simulink model "BiomT1_NOPROP_Model"  (R2023b)
settings: Solver=VariableStepAuto  StartTime=0.0  StopTime=100.0  RelTol=1e-3
values from neighbouring files (symbols this model uses):
  g = 9.81    [initialize_model.m]
  inertiaGeom = load_inertiaGeom()    [computeAeroFM.m]    (also in initialize_model.m)
  x0 = [0 0 zbar u0 v0 w0 0 0 0 0 0 0]    [FlightPerf.m]    (also in initialize_model.m)
libraries: aerolibasang x2, shared6dof x1, aerolibatmos2 x1
settings Model: Creator=sherpa  LastModifiedBy=sudip
settings SolverCC: AlgebraicLoopSolver=TrustRegion
settings OptimizationCC: ReuseModelBlockBuffer=off
settings DebuggingCC: UnconnectedInputMsg=warning  UnconnectedOutputMsg=warning  UnconnectedLineMsg=warning
settings ModelReferenceCC: EnableRefExpFcnMdlSchedulingChecks=on
settings RTWCC: DLArmComputeVersion=19.05

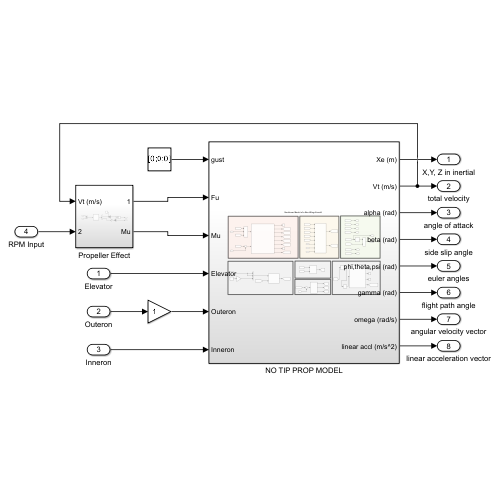
[thumbnail: Simulink's stored preview of the top-level diagram]
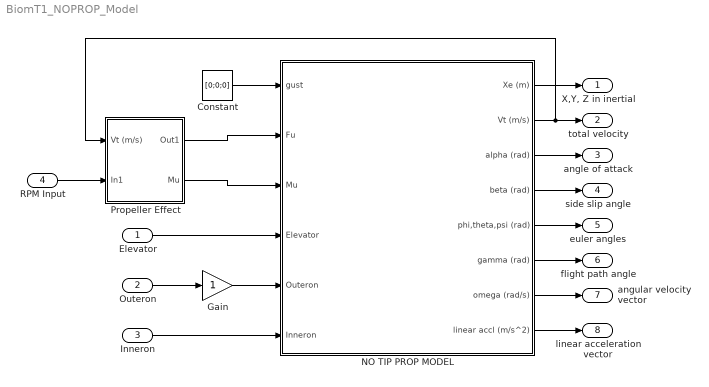
== system BiomT1_NOPROP_Model ==
  Elevator : Inport
  Outeron : Inport  Port=2
  Inneron : Inport  Port=3
  RPM Input : Inport  Port=4
  Constant : Constant  Value=[0;0;0]
  Gain : Gain
  NO TIP PROP MODEL : Subsystem
  Propeller Effect : Subsystem
  "X,Y, Z in inertial" : Outport
  total velocity : Outport  Port=2
  angle of attack : Outport  Port=3
  side slip angle : Outport  Port=4
  euler angles : Outport  Port=5
  flight path angle : Outport  Port=6
  angular velocity vector : Outport  Port=7
  linear acceleration vector : Outport  Port=8
  wires:
  NO TIP PROP MODEL/1(Xe (m)) -> "X,Y, Z in inertial"/1
  NO TIP PROP MODEL/2(Vt (m/s)) -> Propeller Effect/1(Vt (m/s)), total velocity/1
  NO TIP PROP MODEL/3(alpha (rad)) -> angle of attack/1
  NO TIP PROP MODEL/4(beta (rad)) -> side slip angle/1
  NO TIP PROP MODEL/6(gamma (rad)) -> flight path angle/1
  NO TIP PROP MODEL/7(omega (rad/s)) -> angular velocity vector/1
  NO TIP PROP MODEL/8(linear accl (m/s^2)) -> linear acceleration vector/1
  NO TIP PROP MODEL/5(phi,theta,psi (rad)) -> euler angles/1
  Constant/1 -> NO TIP PROP MODEL/1(gust)
  Outeron/1 -> Gain/1
  Inneron/1 -> NO TIP PROP MODEL/6(Inneron)
  Propeller Effect/1(Out1) -> NO TIP PROP MODEL/2(Fu)
  RPM Input/1 -> Propeller Effect/2(In1)
  Propeller Effect/2(Mu) -> NO TIP PROP MODEL/3(Mu)
  Gain/1 -> NO TIP PROP MODEL/5(Outeron)
  Elevator/1 -> NO TIP PROP MODEL/4("Elevator ")

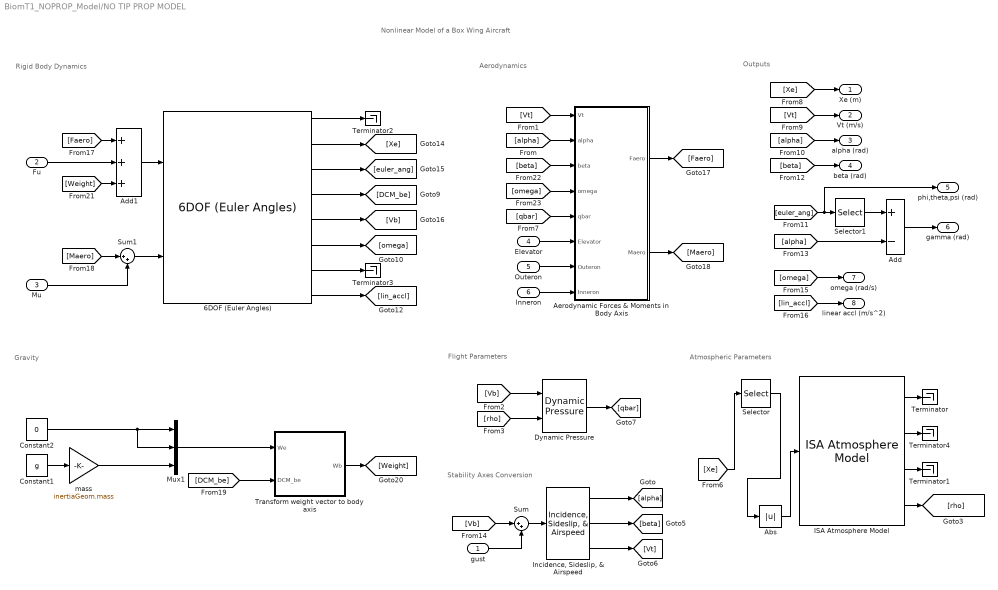
== system BiomT1_NOPROP_Model/NO TIP PROP MODEL ==
  note: Gravity
  note: Nonlinear Model of a Box Wing Aircraft
  note: Aerodynamics
  note: Outputs
  note: Rigid Body Dynamics
  note: Stability Axes Conversion
  note: Atmospheric Parameters
  note: Flight Parameters
  gust : Inport  PortDimensions=3
  Fu : Inport  Port=2  PortDimensions=3
  Mu : Inport  Port=3  PortDimensions=3
  "Elevator " : Inport  Port=4
  Outeron : Inport  Port=5
  Inneron : Inport  Port=6
  6DOF (Euler Angles) : shared6dof/6DOF (Euler Angles)  units=Metric (MKS)  mtype=Fixed  rep=Euler Angles  xme_0=x0(1:3)  Vm_0=x0(4:6)  eul_0=x0(7:9)  pm_0=x0(10:12)  mass_0=inertiaGeom.mass  mass_e=0.5  mass_f=2.0  inertia=inertiaGeom.inertiaMatrix  inertia_e=eye(3)  inertia_f=2*eye(3)  k_quat=1.0  vre_flag=on  abi_flag=off  aMode=0  xme_statename={'Xe','Ye','Ze'}  Vm_statename={'U','v','w'}  eul_statename={'phi','theta','psi'}  quat_statename=''  pm_statename={'p','q','r'}  mass_statename=''
  Abs : Abs  SaturateOnIntegerOverflow=off
  Add : Sum  Inputs=+-
  Add1 : Sum  Inputs=+++
  Aerodynamic Forces & Moments in Body Axis : Subsystem
  Constant1 : Constant  Value=g
  Constant2 : Constant  Value=0
  Dynamic Pressure : aerolibasang/Dynamic Pressure
  ISA Atmosphere Model : aerolibatmos2/ISA Atmosphere Model  useExtended=off  action=Warning  custom=off  viscosityOut=off  g=9.80665  gamma=1.4  R=287.0531  L=0.0065  h_trop=11000  h_strat=20000  rho0=1.225  P0=101325  T0=288.15  h0=0
  "Incidence, Sideslip, & Airspeed" : aerolibasang/Incidence, Sideslip, & Airspeed
  Mux1 : Mux  Inputs=3
  Selector : Selector  InputPortWidth=3  IndexOptions=Index vector (dialog)  Indices=3  OutputSizes=1
  Selector1 : Selector  InputPortWidth=3  IndexOptions=Index vector (dialog)  Indices=2  OutputSizes=1
  Sum : Sum  Inputs=|++
  Sum1 : Sum  Inputs=|++
  Terminator{,1..4} (5 alike) : Terminator
  Transform weight vector to body axis : MATLAB Function  TreatAsAtomicUnit=on
  mass : Gain  Gain=inertiaGeom.mass
  Xe (m) : Outport
  Vt (m/s) : Outport  Port=2
  alpha (rad) : Outport  Port=3
  beta (rad) : Outport  Port=4
  phi,theta,psi (rad) : Outport  Port=5
  gamma (rad) : Outport  Port=6
  omega (rad/s) : Outport  Port=7
  linear accl (m/s^2) : Outport  Port=8
  wires:
  [Xe] -> Selector/1
  [beta] -> beta (rad)/1
  "Incidence, Sideslip, & Airspeed"/3 -> [Vt]
  ISA Atmosphere Model/3 -> Terminator1/1
  ISA Atmosphere Model/1 -> Terminator/1
  ISA Atmosphere Model/4 -> [rho]
  [rho] -> Dynamic Pressure/2
  6DOF (Euler Angles)/3 -> [euler_ang]
  [lin_accl] -> linear accl (m/s^2)/1
  [alpha] -> alpha (rad)/1
  ISA Atmosphere Model/2 -> Terminator4/1
  [Vb] -> Dynamic Pressure/1
  6DOF (Euler Angles)/2 -> [Xe]
  Add/1 -> gamma (rad)/1
  [Vt] -> Vt (m/s)/1
  6DOF (Euler Angles)/7 -> Terminator3/1
  "Incidence, Sideslip, & Airspeed"/2 -> [beta]
  Selector1/1 -> Add/1
  6DOF (Euler Angles)/8 -> [lin_accl]
  6DOF (Euler Angles)/1 -> Terminator2/1
  6DOF (Euler Angles)/6 -> [omega]
  6DOF (Euler Angles)/4 -> [DCM_be]
  "Incidence, Sideslip, & Airspeed"/1 -> [alpha]
  [alpha] -> Add/2
  6DOF (Euler Angles)/5 -> [Vb]
  [euler_ang] -> phi,theta,psi (rad)/1, Selector1/1
  [omega] -> omega (rad/s)/1
  Dynamic Pressure/1 -> [qbar]
  [Xe] -> Xe (m)/1
  Constant1/1 -> mass/1
  mass/1 -> Mux1/3
  Mux1/1 -> Transform weight vector to body axis/1(We)
  Transform weight vector to body axis/1(Wb) -> [Weight]
  [DCM_be] -> Transform weight vector to body axis/2(DCM_be)
  Constant2/1 -> Mux1/2, Mux1/1
  [Faero] -> Add1/1
  Fu/1 -> Add1/2
  [Weight] -> Add1/3
  Add1/1 -> 6DOF (Euler Angles)/1
  [alpha] -> Aerodynamic Forces & Moments in Body Axis/2(alpha)
  [qbar] -> Aerodynamic Forces & Moments in Body Axis/5(qbar)
  Aerodynamic Forces & Moments in Body Axis/1(Faero) -> [Faero]
  Aerodynamic Forces & Moments in Body Axis/2(Maero) -> [Maero]
  [omega] -> Aerodynamic Forces & Moments in Body Axis/4(omega)
  [beta] -> Aerodynamic Forces & Moments in Body Axis/3(beta)
  [Vt] -> Aerodynamic Forces & Moments in Body Axis/1(Vt)
  [Vb] -> Sum/1
  gust/1 -> Sum/2
  Sum1/1 -> 6DOF (Euler Angles)/2
  [Maero] -> Sum1/1
  Mu/1 -> Sum1/2
  "Elevator "/1 -> Aerodynamic Forces & Moments in Body Axis/6("Elevator ")
  Selector/1 -> Abs/1
  Abs/1 -> ISA Atmosphere Model/1
  Outeron/1 -> Aerodynamic Forces & Moments in Body Axis/7(Outeron)
  Inneron/1 -> Aerodynamic Forces & Moments in Body Axis/8(Inneron)
  Sum/1 -> "Incidence, Sideslip, & Airspeed"/1

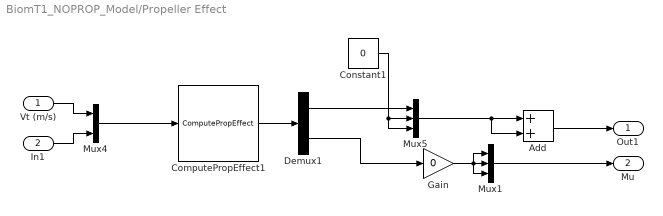
== system BiomT1_NOPROP_Model/Propeller Effect ==
  Vt (m/s) : Inport
  In1 : Inport  Port=2
  Add : Sum
  ComputePropEffect1 : MATLABFcn  MATLABFcn=ComputePropEffect  OutputDimensions=2  OutputSignalType=real
  Constant1 : Constant  Value=0
  Demux1 : Demux  Outputs=2
  Gain : Gain  Gain=0
  Mux1 : Mux  Inputs=3
  Mux4 : Mux  Inputs=2
  Mux5 : Mux  Inputs=3
  Out1 : Outport
  Mu : Outport  Port=2
  wires:
  Demux1/1 -> Mux5/1
  In1/1 -> Mux4/2
  Vt (m/s)/1 -> Mux4/1
  Constant1/1 -> Mux5/3, Mux5/2
  ComputePropEffect1/1 -> Demux1/1
  Mux5/1 -> Add/2, Add/1
  Mux4/1 -> ComputePropEffect1/1
  Add/1 -> Out1/1
  Demux1/2 -> Gain/1
  Gain/1 -> Mux1/3, Mux1/2, Mux1/1
  Mux1/1 -> Mu/1

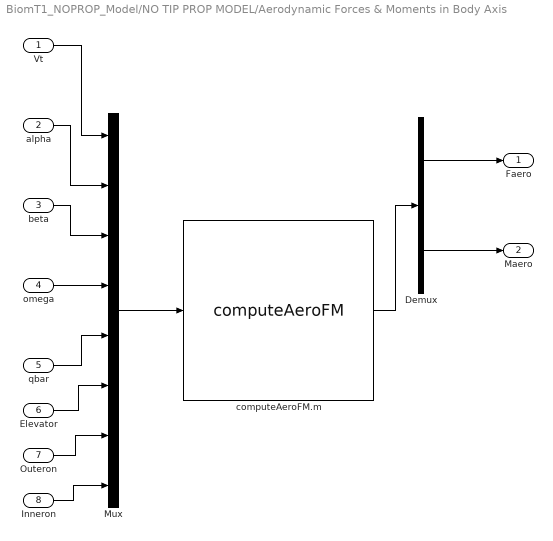
== system BiomT1_NOPROP_Model/NO TIP PROP MODEL/Aerodynamic Forces & Moments in Body Axis ==
  Vt : Inport
  alpha : Inport  Port=2
  beta : Inport  Port=3
  omega : Inport  Port=4
  qbar : Inport  Port=5
  "Elevator " : Inport  Port=6
  Outeron : Inport  Port=7
  Inneron : Inport  Port=8
  Demux : Demux  Outputs=2
  Mux : Mux  Inputs=8
  computeAeroFM.m : MATLABFcn  MATLABFcn=computeAeroFM  OutputDimensions=6  OutputSignalType=real
  Faero : Outport  PortDimensions=3
  Maero : Outport  Port=2  PortDimensions=3
  wires:
  Mux/1 -> computeAeroFM.m/1
  computeAeroFM.m/1 -> Demux/1
  Demux/1 -> Faero/1
  Demux/2 -> Maero/1
  qbar/1 -> Mux/5
  Vt/1 -> Mux/1
  omega/1 -> Mux/4
  beta/1 -> Mux/3
  alpha/1 -> Mux/2
  "Elevator "/1 -> Mux/6
  Outeron/1 -> Mux/7
  Inneron/1 -> Mux/8

== matlab function BiomT1_NOPROP_Model/NO TIP PROP MODEL/Transform weight vector to body axis ==
  data: We input; Wb output; DCM_be input
function Wb = fcn(We,DCM_be)
Wb = DCM_be'*We; % Weight in body coordinate system.
